simulink model "Modelka_1"  (Simulink 4.00)
settings: Solver=ode45  StartTime=0.0  StopTime=10.0  RelTol=1e-3
settings Model: LastModifiedBy=user

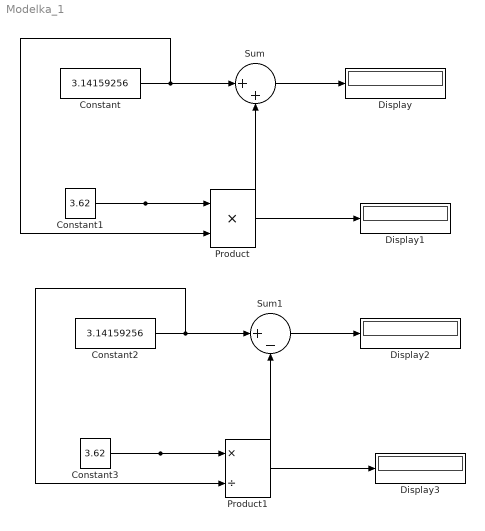
== system Modelka_1 ==
  Constant : Constant  Value=3.14159256
  Constant1 : Constant  Value=3.62
  Constant2 : Constant  Value=3.14159256
  Constant3 : Constant  Value=3.62
  Display{,1..3} (4 alike) : Display
      settings: Format=short
  Product : Product  Inputs=2  Multiplication=Element-wise(.*)  SaturateOnIntegerOverflow=on
  Product1 : Product  Inputs=*/  Multiplication=Element-wise(.*)  SaturateOnIntegerOverflow=on
  Sum : Sum  Inputs=|++  SaturateOnIntegerOverflow=on
  Sum1 : Sum  Inputs=|+-  SaturateOnIntegerOverflow=on
  wires:
  Constant/1 -> Sum/1, Product/2
  Constant1/1 -> Product/1, Sum/2
  Sum/1 -> Display/1
  Product/1 -> Display1/1
  Constant2/1 -> Sum1/1, Product1/2
  Constant3/1 -> Product1/1, Sum1/2
  Sum1/1 -> Display2/1
  Product1/1 -> Display3/1
